simulink model "DTCSMARTGIRD"  (R2025b)
settings: Solver=FixedStepDiscrete  StartTime=0.0  StopTime=10.0  FixedStep=1e-4  RelTol=1e-3
libraries: simulink x1
settings Model: Creator=PRANAV  LastModifiedBy=PRANAV

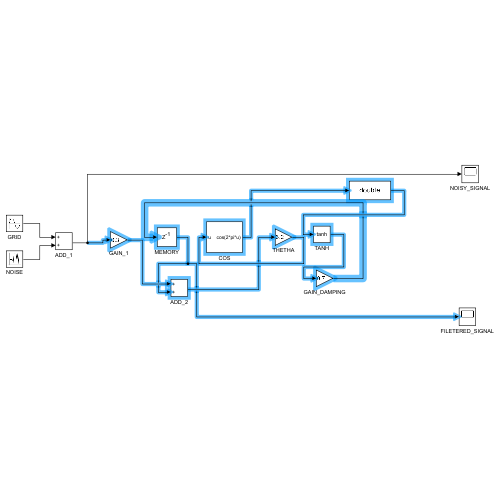
[thumbnail: Simulink's stored preview of the top-level diagram]
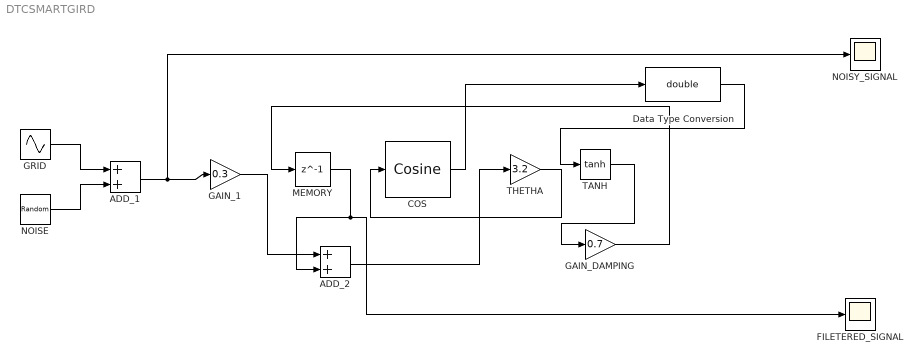
== system DTCSMARTGIRD ==
  ADD_1 : Sum
  ADD_2 : Sum
  COS : simulink/Lookup Tables/Cosine  Formula=cos(2*pi*u)  NumDataPoints=(2^5)+1  OutputWordLength=16  InternalRulePriority=Speed
  Data Type Conversion : DataTypeConversion  OutDataTypeStr=double  SaturateOnIntegerOverflow=off  RndMeth=Floor
  FILETERED_SIGNAL : Scope
      settings: ActiveDisplayYMinimum=-8.1860339827941555  ActiveDisplayYMaximum=16.247234993274631
  GAIN_1 : Gain  Gain=0.3
  GAIN_DAMPING : Gain  Gain=0.7
  GRID : Sin  Frequency=2*pi*50  SampleTime=0
  MEMORY : Delay  DelayLength=1
  NOISE : RandomNumber  SampleTime=0.1
  NOISY_SIGNAL : Scope
      settings: ActiveDisplayYMinimum=-4.29550984403958  ActiveDisplayYMaximum=3.8311634537908086
  TANH : Trigonometry  Operator=tanh
  THETHA : Gain  Gain=3.2
  wires:
  GRID/1 -> ADD_1/1
  NOISE/1 -> ADD_1/2
  ADD_1/1 -> NOISY_SIGNAL/1, GAIN_1/1
  GAIN_1/1 -> ADD_2/1
  MEMORY/1 -> ADD_2/2, FILETERED_SIGNAL/1
  ADD_2/1 -> THETHA/1
  THETHA/1 -> COS/1
  TANH/1 -> GAIN_DAMPING/1
  GAIN_DAMPING/1 -> MEMORY/1
  COS/1 -> Data Type Conversion/1
  Data Type Conversion/1 -> TANH/1
